simulink model "sm_tractor_row_crop"  (R2024b)
settings: Solver=ode23t  StartTime=0.0  StopTime=20  FixedStep=1/1000  MaxStep=0.2  RelTol=1e-3  AbsTol=1e-3  EnableMultiTasking=on
PostLoadFcn:
  | sm_tractor_row_crop_config_maneuver(bdroot,VehicleData,'stepsteer');
StartFcn:
  | tic
StopFcn:
  | Elapsed_Sim_Time = toc;
undefined symbols (not defined in the file): FL, FR, HMPST, InitVehicle, Maneuver, RL, RR, SceneData, targetSpeed, VehicleData, X, Y, Z
libraries: sm_lib x121, sm_vehicle_utilities_lib x41, fl_lib x15, nesl_utility x14, simulink x3, sm_tractor_row_crop_lib x3, sm_tractor_row_crop_lib_vnts x2, Driver_Long_Lat_Stanley x1, Maneuver_Get_Pose x1
(part 2 of 4)

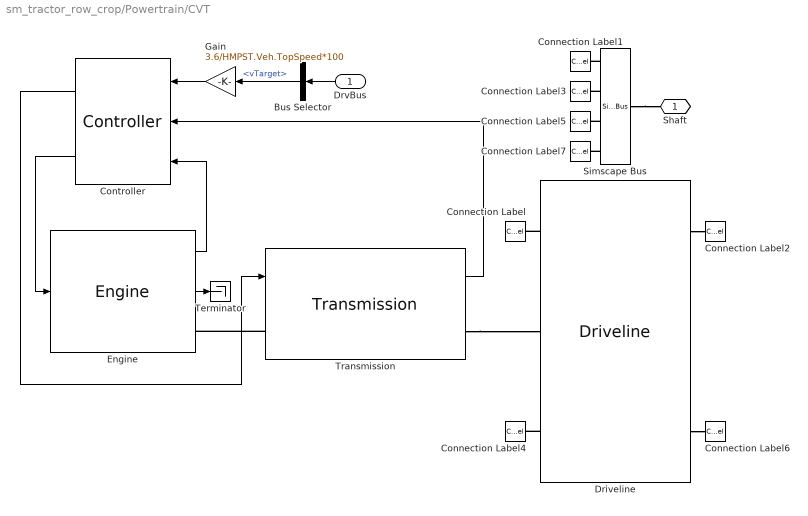
== system sm_tractor_row_crop/Powertrain/CVT ==
  DrvBus : Inport
  Bus Selector : BusSelector  OutputSignals=Reference.vTarget
  Connection Label : ConnectionLabel  Label=FL
  Connection Label1 : ConnectionLabel  Label=FL
  Connection Label2 : ConnectionLabel  Label=FR
  Connection Label3 : ConnectionLabel  Label=FR
  Connection Label4 : ConnectionLabel  Label=RL
  Connection Label5 : ConnectionLabel  Label=RL
  Connection Label6 : ConnectionLabel  Label=RR
  Connection Label7 : ConnectionLabel  Label=RR
  Controller : sm_tractor_row_crop_lib/Controller  SystemSampleTime=-1  VariantActivationTime=update diagram  AllowFlexibleInterface=on  Latency=0  AutoFrameSizeCalculation=off
  Driveline : sm_tractor_row_crop_lib/Driveline  SystemSampleTime=-1  VariantActivationTime=update diagram  AllowFlexibleInterface=on  Latency=0  AutoFrameSizeCalculation=off
  Engine : sm_tractor_row_crop_lib_vnts/Engine  SystemSampleTime=-1  VariantControl=Choice  LabelModeActiveChoice=Droop  VariantActivationTime=update diagram  AllowFlexibleInterface=on  Latency=0  AutoFrameSizeCalculation=off
      settings: AttributesFormatString=%<LabelModeActiveChoice>
  Gain : Gain  Gain=3.6/HMPST.Veh.TopSpeed*100
  Simscape Bus : SimscapeBus  HierarchyStrings=FL;FR;RL;RR
  Terminator : Terminator
  Transmission : sm_tractor_row_crop_lib_vnts/Transmission  SystemSampleTime=-1  VariantControl=Choice  LabelModeActiveChoice=Hydrostatic  VariantActivationTime=update diagram  AllowFlexibleInterface=on  Latency=0  AutoFrameSizeCalculation=off
      settings: AttributesFormatString=%<LabelModeActiveChoice>
  Shaft : PMIOPort  Side=Right
  wires:
  Engine/2 -> Terminator/1
  Transmission/1 -> Controller/2
  Controller/1 -> Transmission/1
  Controller/2 -> Engine/1
  Engine/1 -> Controller/3
  Bus Selector/1 -> Gain/1  "<vTarget>"
  Gain/1 -> Controller/1
  DrvBus/1 -> Bus Selector/1
  connections:
  Transmission/RConn1 -- Driveline/LConn2
  Simscape Bus/RConn1 -- Shaft/RConn1
  Transmission/LConn1 -- Engine/RConn1
  Simscape Bus/LConn2 -- Connection Label3/LConn1
  Simscape Bus/LConn1 -- Connection Label1/LConn1
  Simscape Bus/LConn4 -- Connection Label7/LConn1
  Simscape Bus/LConn3 -- Connection Label5/LConn1
  Driveline/LConn1 -- Connection Label4/LConn1
  Driveline/LConn3 -- Connection Label/LConn1
  Driveline/RConn1 -- Connection Label6/LConn1
  Driveline/RConn3 -- Connection Label2/LConn1

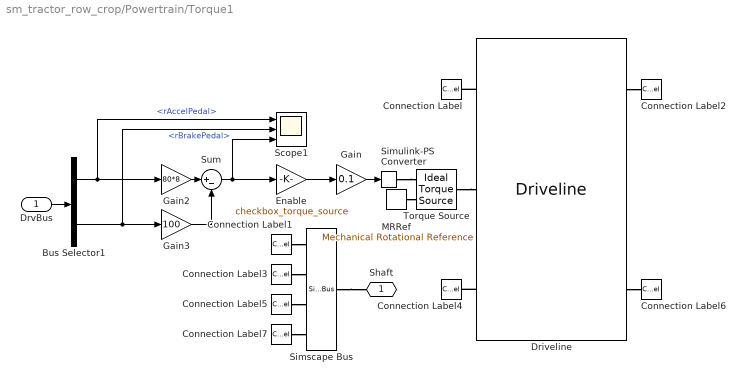
== system sm_tractor_row_crop/Powertrain/Torque1 ==
  DrvBus : Inport
  Bus Selector1 : BusSelector  OutputSignals=rAccelPedal,rBrakePedal
  Connection Label : ConnectionLabel  Label=FL
  Connection Label1 : ConnectionLabel  Label=FL
  Connection Label2 : ConnectionLabel  Label=FR
  Connection Label3 : ConnectionLabel  Label=FR
  Connection Label4 : ConnectionLabel  Label=RL
  Connection Label5 : ConnectionLabel  Label=RL
  Connection Label6 : ConnectionLabel  Label=RR
  Connection Label7 : ConnectionLabel  Label=RR
  Driveline : sm_tractor_row_crop_lib/Driveline  SystemSampleTime=-1  VariantActivationTime=update diagram  AllowFlexibleInterface=on  Latency=0  AutoFrameSizeCalculation=off
  Enable : Gain  Gain=checkbox_torque_source
  Gain : Gain  Gain=0.1
  Gain2 : Gain  Gain=80*8
  Gain3 : Gain  Gain=100
  MRRef : fl_lib/Mechanical/Rotational Elements/Mechanical Rotational Reference
  Scope1 : Scope  NumInputPorts=3
  Simscape Bus : SimscapeBus  HierarchyStrings=FL;FR;RL;RR
  Simulink-PS Converter : nesl_utility/Simulink-PS Converter  PhysicalDomain=network_engine_domain  SubClassName=ps_input  LeftPortType=input  RightPortType=output  PseudoPeriodic=off  Frequencies=[]  NoiseDistribution=none  NoiseParameters=[]  Unit=1  AffineConversion=off  FilteringAndDerivatives=provide  SimscapeFilterOrder=1  InputFilterTimeConstant=0.001  UdotUserProvided=0
  Sum : Sum  Inputs=|+-
  Torque Source : fl_lib/Mechanical/Mechanical Sources/Ideal Torque Source
  Shaft : PMIOPort  Side=Right
  wires:
  Sum/1 -> Scope1/3, Enable/1
  DrvBus/1 -> Bus Selector1/1
  Bus Selector1/2 -> Scope1/2, Gain3/1  "<rBrakePedal>"
  Gain3/1 -> Sum/2
  Gain2/1 -> Sum/1
  Bus Selector1/1 -> Scope1/1, Gain2/1  "<rAccelPedal>"
  Gain/1 -> Simulink-PS Converter/1
  Enable/1 -> Gain/1
  connections:
  Driveline/RConn3 -- Connection Label2/LConn1
  Driveline/LConn3 -- Connection Label/LConn1
  Driveline/RConn1 -- Connection Label6/LConn1
  Driveline/LConn1 -- Connection Label4/LConn1
  Simscape Bus/RConn1 -- Shaft/RConn1
  MRRef/LConn1 -- Torque Source/RConn2
  Torque Source/LConn1 -- Driveline/LConn2
  Simulink-PS Converter/RConn1 -- Torque Source/RConn1
  Connection Label1/LConn1 -- Simscape Bus/LConn1
  Connection Label3/LConn1 -- Simscape Bus/LConn2
  Connection Label5/LConn1 -- Simscape Bus/LConn3
  Connection Label7/LConn1 -- Simscape Bus/LConn4

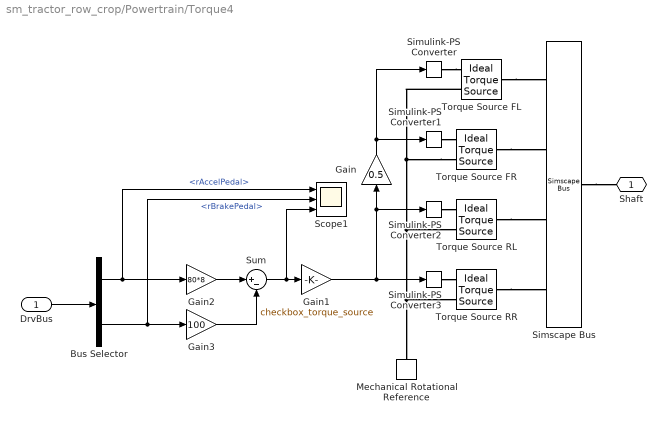
== system sm_tractor_row_crop/Powertrain/Torque4 ==
  DrvBus : Inport
  Bus Selector : BusSelector  OutputSignals=rAccelPedal,rBrakePedal
  Gain : Gain  Gain=0.5
  Gain1 : Gain  Gain=checkbox_torque_source
  Gain2 : Gain  Gain=80*8
  Gain3 : Gain  Gain=100
  Mechanical Rotational Reference : fl_lib/Mechanical/Rotational Elements/Mechanical Rotational Reference
  Scope1 : Scope  NumInputPorts=3
  Simscape Bus : SimscapeBus  HierarchyStrings=FL;FR;RL;RR
  Simulink-PS Converter{,1..3} (4 alike) : nesl_utility/Simulink-PS Converter  PhysicalDomain=network_engine_domain  SubClassName=ps_input  LeftPortType=input  RightPortType=output  PseudoPeriodic=off  Frequencies=[]  NoiseDistribution=none  NoiseParameters=[]  Unit=1  AffineConversion=off  FilteringAndDerivatives=provide  SimscapeFilterOrder=1  InputFilterTimeConstant=0.001  UdotUserProvided=0
  Sum : Sum  Inputs=|+-
  Torque Source FL : fl_lib/Mechanical/Mechanical Sources/Ideal Torque Source
  Torque Source FR : fl_lib/Mechanical/Mechanical Sources/Ideal Torque Source
  Torque Source RL : fl_lib/Mechanical/Mechanical Sources/Ideal Torque Source
  Torque Source RR : fl_lib/Mechanical/Mechanical Sources/Ideal Torque Source
  Shaft : PMIOPort  Side=Right
  wires:
  Bus Selector/1 -> Scope1/1, Gain2/1  "<rAccelPedal>"
  DrvBus/1 -> Bus Selector/1
  Sum/1 -> Scope1/3, Gain1/1
  Bus Selector/2 -> Scope1/2, Gain3/1  "<rBrakePedal>"
  Gain2/1 -> Sum/1
  Gain3/1 -> Sum/2
  Gain1/1 -> Simulink-PS Converter3/1, Simulink-PS Converter2/1, Gain/1
  Gain/1 -> Simulink-PS Converter1/1, Simulink-PS Converter/1
  connections:
  Torque Source FR/RConn2 -- Mechanical Rotational Reference/LConn1 -- Torque Source RR/RConn2 -- Torque Source RL/RConn2 -- Torque Source FL/RConn2
  Simulink-PS Converter3/RConn1 -- Torque Source RR/RConn1
  Simulink-PS Converter2/RConn1 -- Torque Source RL/RConn1
  Simulink-PS Converter1/RConn1 -- Torque Source FR/RConn1
  Simulink-PS Converter/RConn1 -- Torque Source FL/RConn1
  Torque Source RR/LConn1 -- Simscape Bus/LConn4
  Torque Source RL/LConn1 -- Simscape Bus/LConn3
  Torque Source FR/LConn1 -- Simscape Bus/LConn2
  Torque Source FL/LConn1 -- Simscape Bus/LConn1
  Simscape Bus/RConn1 -- Shaft/RConn1

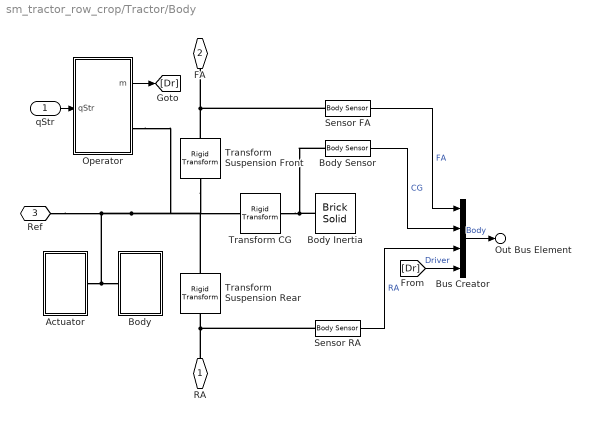
== system sm_tractor_row_crop/Tractor/Body ==
  qStr : Inport
  Actuator : Subsystem
  Body : Subsystem
  Body Inertia : sm_lib/Body Elements/Brick Solid  BrickDimensions=[0.1 0.1 0.1]  BrickDimensionsUnits=m  ExportEntireGeometry=off  InertiaType=Custom  BasedOnType=Density  Density=1000  DensityUnits=kg/(m^3)  Mass=mBody  MassUnits=kg  CenterOfMass=[0 0 0]  CenterOfMassUnits=m  MomentsOfInertia=JBody  MomentsOfInertiaUnits=kg*m^2  ProductsOfInertia=[0 0 0]  ProductsOfInertiaUnits=kg*m^2  GraphicType=FromGeometry  MarkerShape=Sphere  MarkerSize=10  GraphicVisPropType=SimpleVisualProperties  GraphicDiffuseColor=[0.4 0.6 1.0]  GraphicOpacity=1.0  GraphicSpecularColor=[0.5 0.5 0.5 1.0]  GraphicAmbientColor=[0.15 0.15 0.15 1.0]  GraphicEmissiveColor=[0.0 0.0 0.0 1.0]  GraphicShininess=75  DoExposeReferenceFrame=on  SerializedFrames=<Frames/>
  Body Sensor : sm_vehicle_utilities_lib/Body Sensor  offset_body_sensor=[0 0 0]
  Bus Creator : BusCreator  Inputs=4
  Operator : Subsystem  mask{popup_operator=None}
      mask prompts: popup_operator "Operator Type"
      mask init:
      | bh = gcb;
      | op_type = get_param(bh,'popup_operator');
      | switch op_type
      |     case 'None'
      |         set_param([bh '/Operator'],'popup_operator','None');
      |         set_param([bh '/Suspension'],'popup_suspension','None');
      |     case 'Human, Rigid Seat'
      |         set_param([bh '/Operator'],'popup_operator','Human');
      |         set_param([bh '/Suspension'],'popup_suspension','None');
      |     case 'Human, Suspension'
      |         set_param([bh '/Operator'],'popup_operator','Human');
      |         set_param([bh '/Suspension'],'popup_suspension','Heave Linear');
      | end
      settings: AttributesFormatString=%<popup_operator>
      mask TypeOptions popup_operator: None | Human, Rigid Seat | Human, Suspension
  Sensor FA : sm_vehicle_utilities_lib/Body Sensor  offset_body_sensor=[0 0 0]
  Sensor RA : sm_vehicle_utilities_lib/Body Sensor  offset_body_sensor=[0 0 0]
  Transform CG : sm_lib/Frames and Transforms/Rigid Transform  RotationMethod=None  FollAlignAxisA=+X  BaseAlignAxisA=+Y  FollAlignAxisB=+Y  BaseAlignAxisB=+Z  RotationStandardAxis=+Z  RotationAngle=0  RotationAngleUnits=deg  RotationArbitraryAxis=[0 0 1]  RotationSequenceAxes=FollowerAxes  RotationSequence=XYX  RotationSequenceAngles=[0 0 0]  RotationSequenceAnglesUnits=deg  RotationMatrix=[1 0 0; 0 1 0; 0 0 1]  Quaternion=[1 0 0 0]  TranslationMethod=Cartesian  TranslationCartesianOffset=xyzRefToCG  TranslationCartesianOffsetUnits=m  TranslationStandardAxis=+Z  TranslationStandardOffset=0  TranslationStandardOffsetUnits=m  TranslationROffset=0  TranslationROffsetUnits=m  TranslationThetaOffset=0  TranslationThetaOffsetUnits=deg  TranslationZOffset=0  TranslationZOffsetUnits=m
  Transform Suspension Front : sm_lib/Frames and Transforms/Rigid Transform  RotationMethod=None  FollAlignAxisA=+X  BaseAlignAxisA=+Y  FollAlignAxisB=+Y  BaseAlignAxisB=+Z  RotationStandardAxis=+Z  RotationAngle=0  RotationAngleUnits=deg  RotationArbitraryAxis=[0 0 1]  RotationSequenceAxes=FollowerAxes  RotationSequence=XYX  RotationSequenceAngles=[0 0 0]  RotationSequenceAnglesUnits=deg  RotationMatrix=[1 0 0; 0 1 0; 0 0 1]  Quaternion=[1 0 0 0]  TranslationMethod=StandardAxis  TranslationCartesianOffset=[0 0 0]  TranslationCartesianOffsetUnits=m  TranslationStandardAxis=+X  TranslationStandardOffset=xRefToFA  TranslationStandardOffsetUnits=m  TranslationROffset=0  TranslationROffsetUnits=m  TranslationThetaOffset=0  TranslationThetaOffsetUnits=deg  TranslationZOffset=0  TranslationZOffsetUnits=m
  Transform Suspension Rear : sm_lib/Frames and Transforms/Rigid Transform  RotationMethod=None  FollAlignAxisA=+X  BaseAlignAxisA=+Y  FollAlignAxisB=+Y  BaseAlignAxisB=+Z  RotationStandardAxis=+Z  RotationAngle=0  RotationAngleUnits=deg  RotationArbitraryAxis=[0 0 1]  RotationSequenceAxes=FollowerAxes  RotationSequence=XYX  RotationSequenceAngles=[0 0 0]  RotationSequenceAnglesUnits=deg  RotationMatrix=[1 0 0; 0 1 0; 0 0 1]  Quaternion=[1 0 0 0]  TranslationMethod=StandardAxis  TranslationCartesianOffset=[0 0 0]  TranslationCartesianOffsetUnits=m  TranslationStandardAxis=+X  TranslationStandardOffset=xRefToRA  TranslationStandardOffsetUnits=m  TranslationROffset=0  TranslationROffsetUnits=m  TranslationThetaOffset=0  TranslationThetaOffsetUnits=deg  TranslationZOffset=0  TranslationZOffsetUnits=m
  RA : PMIOPort  Side=Left
  FA : PMIOPort  Port=2  Side=Right
  Ref : PMIOPort  Port=3  Side=Right
  Out Bus Element : Outport  PortName=m  Element=Body
  wires:
  Body Sensor/1 -> Bus Creator/2  "CG"
  Sensor FA/1 -> Bus Creator/1  "FA"
  Sensor RA/1 -> Bus Creator/3  "RA"
  Bus Creator/1 -> Out Bus Element/1  "Body"
  [Dr] -> Bus Creator/4  "Driver"
  qStr/1 -> Operator/1(qStr)
  Operator/1(m) -> [Dr]
  connections:
  RA/RConn1 -- Transform Suspension Rear/RConn1 -- Sensor RA/LConn1
  Actuator/LConn1 -- Body/RConn1 -- Ref/RConn1 -- Operator/RConn1 -- Transform Suspension Front/LConn1 -- Transform Suspension Rear/LConn1 -- Transform CG/LConn1
  Transform Suspension Front/RConn1 -- FA/RConn1 -- Sensor FA/LConn1
  Transform CG/RConn1 -- Body Inertia/RConn1 -- Body Sensor/LConn1

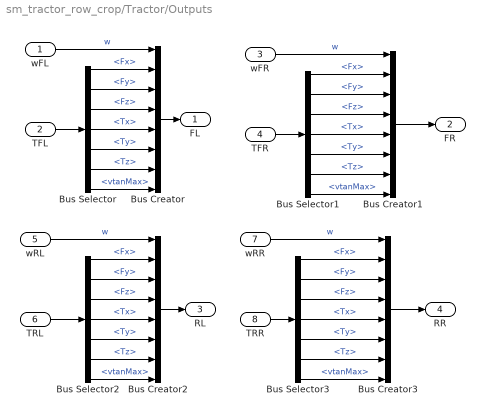
== system sm_tractor_row_crop/Tractor/Outputs ==
  wFL : Inport
  TFL : Inport  Port=2
  wFR : Inport  Port=3
  TFR : Inport  Port=4
  wRL : Inport  Port=5
  TRL : Inport  Port=6
  wRR : Inport  Port=7
  TRR : Inport  Port=8
  Bus Creator{,1..3} (4 alike) : BusCreator  Inputs=8
  Bus Selector{,1..3} (4 alike) : BusSelector  OutputSignals=Fx,Fy,Fz,Tx,Ty,Tz,vtanMax
  FL : Outport
  FR : Outport  Port=2
  RL : Outport  Port=3
  RR : Outport  Port=4
  wires:
  TFL/1 -> Bus Selector/1
  Bus Selector/1 -> Bus Creator/2  "<Fx>"
  Bus Selector/3 -> Bus Creator/4  "<Fz>"
  Bus Selector/4 -> Bus Creator/5  "<Tx>"
  wFL/1 -> Bus Creator/1  "w"
  Bus Selector/2 -> Bus Creator/3  "<Fy>"
  Bus Selector/6 -> Bus Creator/7  "<Tz>"
  Bus Selector/5 -> Bus Creator/6  "<Ty>"
  Bus Creator/1 -> FL/1
  Bus Creator1/1 -> FR/1
  Bus Selector1/5 -> Bus Creator1/6  "<Ty>"
  Bus Selector1/6 -> Bus Creator1/7  "<Tz>"
  Bus Selector1/2 -> Bus Creator1/3  "<Fy>"
  wFR/1 -> Bus Creator1/1  "w"
  Bus Selector1/4 -> Bus Creator1/5  "<Tx>"
  Bus Selector1/3 -> Bus Creator1/4  "<Fz>"
  Bus Selector1/1 -> Bus Creator1/2  "<Fx>"
  TFR/1 -> Bus Selector1/1
  TRR/1 -> Bus Selector3/1
  Bus Selector3/1 -> Bus Creator3/2  "<Fx>"
  Bus Selector3/3 -> Bus Creator3/4  "<Fz>"
  Bus Selector3/4 -> Bus Creator3/5  "<Tx>"
  wRR/1 -> Bus Creator3/1  "w"
  Bus Selector3/2 -> Bus Creator3/3  "<Fy>"
  Bus Selector3/6 -> Bus Creator3/7  "<Tz>"
  Bus Selector3/5 -> Bus Creator3/6  "<Ty>"
  Bus Creator3/1 -> RR/1
  Bus Creator2/1 -> RL/1
  Bus Selector2/5 -> Bus Creator2/6  "<Ty>"
  Bus Selector2/6 -> Bus Creator2/7  "<Tz>"
  Bus Selector2/2 -> Bus Creator2/3  "<Fy>"
  wRL/1 -> Bus Creator2/1  "w"
  Bus Selector2/4 -> Bus Creator2/5  "<Tx>"
  Bus Selector2/3 -> Bus Creator2/4  "<Fz>"
  Bus Selector2/1 -> Bus Creator2/2  "<Fx>"
  TRL/1 -> Bus Selector2/1
  Bus Selector/7 -> Bus Creator/8  "<vtanMax>"
  Bus Selector1/7 -> Bus Creator1/8  "<vtanMax>"
  Bus Selector2/7 -> Bus Creator2/8  "<vtanMax>"
  Bus Selector3/7 -> Bus Creator3/8  "<vtanMax>"

== system sm_tractor_row_crop/Tractor/Revolute Whl FL ==
  Mechanical Rotational Reference : fl_lib/Mechanical/Rotational Elements/Mechanical Rotational Reference
  Multibody-1D Interface : fl_lib/Mechanical/Multibody Interfaces/Rotational Multibody Interface
  PS-Simulink Converter : nesl_utility/PS-Simulink Converter  PhysicalDomain=network_engine_domain  SubClassName=ps_output  LeftPortType=input  RightPortType=output  PseudoPeriodic=off  Frequencies=[]  VectorFormat=inherit  Unit=inherit  AffineConversion=off
  Revolute Joint : sm_lib/Joints/Revolute Joint  JointMode=Normal  CompositeWrenchDir=FollowerOnBase  CompositeWrenchFrame=BaseFrame  SenseConstraintForce=off  SenseConstraintTorque=off  SenseTotalForce=off  SenseTotalTorque=off  PositionTargetSpecify=off  PositionTargetPriority=High  PositionTargetValue=0  PositionTargetValueUnits=deg  VelocityTargetSpecify=on  VelocityTargetPriority=High  VelocityTargetValue=initveh.Wheel.wFL  VelocityTargetValueUnits=rad/s  EquilibriumPosition=0  EquilibriumPositionUnits=rad  SpringStiffness=0  SpringStiffnessUnits=N*m/rad  DampingCoefficient=0  DampingCoefficientUnits=N*m/(rad/s)  LowerLimitSpecify=off  LowerLimitBound=-90  LowerLimitBoundUnits=deg  LowerLimitStiffness=1e4  LowerLimitStiffnessUnits=N*m/deg  LowerLimitDamping=10  LowerLimitDampingUnits=N*m/(deg/s)  LowerLimitTransitionRegionWidth=0.1  LowerLimitTransitionRegionWidthUnits=deg  UpperLimitSpecify=off  UpperLimitBound=90  UpperLimitBoundUnits=deg  UpperLimitStiffness=1e4  UpperLimitStiffnessUnits=N*m/deg  UpperLimitDamping=10  UpperLimitDampingUnits=N*m/(deg/s)  UpperLimitTransitionRegionWidth=0.1  UpperLimitTransitionRegionWidthUnits=deg  TorqueActuationMode=InputTorque  MotionActuationMode=ComputedMotion  SensePosition=off  SenseVelocity=on  SenseAcceleration=off  SenseTorqueForce=off  SenseLowerLimitTorqueForce=off  SenseUpperLimitTorqueForce=off
  B : PMIOPort  Side=Right
  R : PMIOPort  Port=2  Side=Left
  F : PMIOPort  Port=3  Side=Left
  Out Bus Element : Outport  PortName=m  Element=w
  wires:
  PS-Simulink Converter/1 -> Out Bus Element/1
  connections:
  Revolute Joint/LConn2 -- Multibody-1D Interface/LConn1
  Revolute Joint/RConn2 -- PS-Simulink Converter/LConn1 -- Multibody-1D Interface/RConn1
  F/RConn1 -- Revolute Joint/RConn1
  B/RConn1 -- Revolute Joint/LConn1
  Multibody-1D Interface/LConn2 -- Mechanical Rotational Reference/LConn1
  R/RConn1 -- Multibody-1D Interface/RConn2

== system sm_tractor_row_crop/Tractor/Revolute Whl FR ==
  Mechanical Rotational Reference : fl_lib/Mechanical/Rotational Elements/Mechanical Rotational Reference
  Multibody-1D Interface : fl_lib/Mechanical/Multibody Interfaces/Rotational Multibody Interface
  PS-Simulink Converter : nesl_utility/PS-Simulink Converter  PhysicalDomain=network_engine_domain  SubClassName=ps_output  LeftPortType=input  RightPortType=output  PseudoPeriodic=off  Frequencies=[]  VectorFormat=inherit  Unit=inherit  AffineConversion=off
  Revolute Joint : sm_lib/Joints/Revolute Joint  JointMode=Normal  CompositeWrenchDir=FollowerOnBase  CompositeWrenchFrame=BaseFrame  SenseConstraintForce=off  SenseConstraintTorque=off  SenseTotalForce=off  SenseTotalTorque=off  PositionTargetSpecify=off  PositionTargetPriority=High  PositionTargetValue=0  PositionTargetValueUnits=deg  VelocityTargetSpecify=on  VelocityTargetPriority=High  VelocityTargetValue=initveh.Wheel.wFR  VelocityTargetValueUnits=rad/s  EquilibriumPosition=0  EquilibriumPositionUnits=rad  SpringStiffness=0  SpringStiffnessUnits=N*m/rad  DampingCoefficient=0  DampingCoefficientUnits=N*m/(rad/s)  LowerLimitSpecify=off  LowerLimitBound=-90  LowerLimitBoundUnits=deg  LowerLimitStiffness=1e4  LowerLimitStiffnessUnits=N*m/deg  LowerLimitDamping=10  LowerLimitDampingUnits=N*m/(deg/s)  LowerLimitTransitionRegionWidth=0.1  LowerLimitTransitionRegionWidthUnits=deg  UpperLimitSpecify=off  UpperLimitBound=90  UpperLimitBoundUnits=deg  UpperLimitStiffness=1e4  UpperLimitStiffnessUnits=N*m/deg  UpperLimitDamping=10  UpperLimitDampingUnits=N*m/(deg/s)  UpperLimitTransitionRegionWidth=0.1  UpperLimitTransitionRegionWidthUnits=deg  TorqueActuationMode=InputTorque  MotionActuationMode=ComputedMotion  SensePosition=off  SenseVelocity=on  SenseAcceleration=off  SenseTorqueForce=off  SenseLowerLimitTorqueForce=off  SenseUpperLimitTorqueForce=off
  B : PMIOPort  Side=Right
  R : PMIOPort  Port=2  Side=Left
  F : PMIOPort  Port=3  Side=Left
  Out Bus Element : Outport  PortName=m  Element=w
  wires:
  PS-Simulink Converter/1 -> Out Bus Element/1
  connections:
  R/RConn1 -- Multibody-1D Interface/RConn2
  Multibody-1D Interface/LConn2 -- Mechanical Rotational Reference/LConn1
  B/RConn1 -- Revolute Joint/LConn1
  F/RConn1 -- Revolute Joint/RConn1
  PS-Simulink Converter/LConn1 -- Revolute Joint/RConn2 -- Multibody-1D Interface/RConn1
  Revolute Joint/LConn2 -- Multibody-1D Interface/LConn1

== system sm_tractor_row_crop/Tractor/Revolute Whl RL ==
  Mechanical Rotational Reference : fl_lib/Mechanical/Rotational Elements/Mechanical Rotational Reference
  Multibody-1D Interface : fl_lib/Mechanical/Multibody Interfaces/Rotational Multibody Interface
  PS-Simulink Converter : nesl_utility/PS-Simulink Converter  PhysicalDomain=network_engine_domain  SubClassName=ps_output  LeftPortType=input  RightPortType=output  PseudoPeriodic=off  Frequencies=[]  VectorFormat=inherit  Unit=inherit  AffineConversion=off
  Revolute Joint : sm_lib/Joints/Revolute Joint  JointMode=Normal  CompositeWrenchDir=FollowerOnBase  CompositeWrenchFrame=BaseFrame  SenseConstraintForce=off  SenseConstraintTorque=off  SenseTotalForce=off  SenseTotalTorque=off  PositionTargetSpecify=off  PositionTargetPriority=High  PositionTargetValue=0  PositionTargetValueUnits=deg  VelocityTargetSpecify=on  VelocityTargetPriority=High  VelocityTargetValue=initveh.Wheel.wRL  VelocityTargetValueUnits=rad/s  EquilibriumPosition=0  EquilibriumPositionUnits=rad  SpringStiffness=0  SpringStiffnessUnits=N*m/rad  DampingCoefficient=0  DampingCoefficientUnits=N*m/(rad/s)  LowerLimitSpecify=off  LowerLimitBound=-90  LowerLimitBoundUnits=deg  LowerLimitStiffness=1e4  LowerLimitStiffnessUnits=N*m/deg  LowerLimitDamping=10  LowerLimitDampingUnits=N*m/(deg/s)  LowerLimitTransitionRegionWidth=0.1  LowerLimitTransitionRegionWidthUnits=deg  UpperLimitSpecify=off  UpperLimitBound=90  UpperLimitBoundUnits=deg  UpperLimitStiffness=1e4  UpperLimitStiffnessUnits=N*m/deg  UpperLimitDamping=10  UpperLimitDampingUnits=N*m/(deg/s)  UpperLimitTransitionRegionWidth=0.1  UpperLimitTransitionRegionWidthUnits=deg  TorqueActuationMode=InputTorque  MotionActuationMode=ComputedMotion  SensePosition=off  SenseVelocity=on  SenseAcceleration=off  SenseTorqueForce=off  SenseLowerLimitTorqueForce=off  SenseUpperLimitTorqueForce=off
  B : PMIOPort  Side=Right
  R : PMIOPort  Port=2  Side=Left
  F : PMIOPort  Port=3  Side=Left
  Out Bus Element : Outport  PortName=m  Element=w
  wires:
  PS-Simulink Converter/1 -> Out Bus Element/1
  connections:
  R/RConn1 -- Multibody-1D Interface/RConn2
  Multibody-1D Interface/LConn2 -- Mechanical Rotational Reference/LConn1
  B/RConn1 -- Revolute Joint/LConn1
  F/RConn1 -- Revolute Joint/RConn1
  PS-Simulink Converter/LConn1 -- Revolute Joint/RConn2 -- Multibody-1D Interface/RConn1
  Revolute Joint/LConn2 -- Multibody-1D Interface/LConn1

== system sm_tractor_row_crop/Tractor/Revolute Whl RR ==
  Mechanical Rotational Reference : fl_lib/Mechanical/Rotational Elements/Mechanical Rotational Reference
  Multibody-1D Interface : fl_lib/Mechanical/Multibody Interfaces/Rotational Multibody Interface
  PS-Simulink Converter : nesl_utility/PS-Simulink Converter  PhysicalDomain=network_engine_domain  SubClassName=ps_output  LeftPortType=input  RightPortType=output  PseudoPeriodic=off  Frequencies=[]  VectorFormat=inherit  Unit=inherit  AffineConversion=off
  Revolute Joint : sm_lib/Joints/Revolute Joint  JointMode=Normal  CompositeWrenchDir=FollowerOnBase  CompositeWrenchFrame=BaseFrame  SenseConstraintForce=off  SenseConstraintTorque=off  SenseTotalForce=off  SenseTotalTorque=off  PositionTargetSpecify=off  PositionTargetPriority=High  PositionTargetValue=0  PositionTargetValueUnits=deg  VelocityTargetSpecify=on  VelocityTargetPriority=High  VelocityTargetValue=initveh.Wheel.wRR  VelocityTargetValueUnits=rad/s  EquilibriumPosition=0  EquilibriumPositionUnits=rad  SpringStiffness=0  SpringStiffnessUnits=N*m/rad  DampingCoefficient=0  DampingCoefficientUnits=N*m/(rad/s)  LowerLimitSpecify=off  LowerLimitBound=-90  LowerLimitBoundUnits=deg  LowerLimitStiffness=1e4  LowerLimitStiffnessUnits=N*m/deg  LowerLimitDamping=10  LowerLimitDampingUnits=N*m/(deg/s)  LowerLimitTransitionRegionWidth=0.1  LowerLimitTransitionRegionWidthUnits=deg  UpperLimitSpecify=off  UpperLimitBound=90  UpperLimitBoundUnits=deg  UpperLimitStiffness=1e4  UpperLimitStiffnessUnits=N*m/deg  UpperLimitDamping=10  UpperLimitDampingUnits=N*m/(deg/s)  UpperLimitTransitionRegionWidth=0.1  UpperLimitTransitionRegionWidthUnits=deg  TorqueActuationMode=InputTorque  MotionActuationMode=ComputedMotion  SensePosition=off  SenseVelocity=on  SenseAcceleration=off  SenseTorqueForce=off  SenseLowerLimitTorqueForce=off  SenseUpperLimitTorqueForce=off
  B : PMIOPort  Side=Right
  R : PMIOPort  Port=2  Side=Left
  F : PMIOPort  Port=3  Side=Left
  Out Bus Element : Outport  PortName=m  Element=w
  wires:
  PS-Simulink Converter/1 -> Out Bus Element/1
  connections:
  Revolute Joint/LConn2 -- Multibody-1D Interface/LConn1
  Multibody-1D Interface/RConn1 -- Revolute Joint/RConn2 -- PS-Simulink Converter/LConn1
  F/RConn1 -- Revolute Joint/RConn1
  B/RConn1 -- Revolute Joint/LConn1
  Multibody-1D Interface/LConn2 -- Mechanical Rotational Reference/LConn1
  R/RConn1 -- Multibody-1D Interface/RConn2

== system sm_tractor_row_crop/Tractor/Scene ==
  Flat : Subsystem  VariantControl=Flat
  Orchard : Subsystem  VariantControl=Orchard
  Plateau : Subsystem  VariantControl=Plateau
  Rough Road : Subsystem  VariantControl=Rough_Road
  Uneven Road : Subsystem  VariantControl=Uneven_Road
  GFL : PMIOPort  Side=Left
  GFR : PMIOPort  Port=2  Side=Left
  GRL : PMIOPort  Port=3  Side=Left
  GRR : PMIOPort  Port=4  Side=Left
  RFL : PMIOPort  Port=5  Side=Left
  RFR : PMIOPort  Port=6  Side=Left
  RRL : PMIOPort  Port=7  Side=Left
  RRR : PMIOPort  Port=8  Side=Left

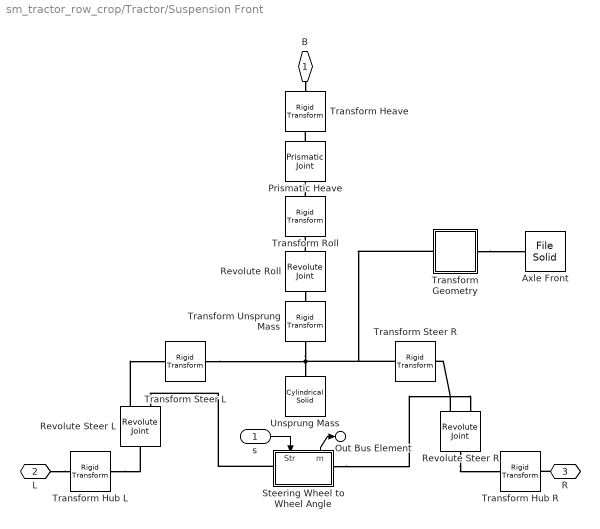
== system sm_tractor_row_crop/Tractor/Suspension Front ==
  s : Inport
  Axle Front : sm_lib/Body Elements/File Solid  ExtGeomFileName=Axle_Front.stl  UnitType=Custom  ExtGeomFileUnits=m  StepReaderType=HEX  ExportConvexHullGeometry=off  InertiaType=PointMass  BasedOnType=Density  Density=1000  DensityUnits=kg/m^3  Mass=0  MassUnits=kg  CenterOfMass=[0 0 0]  CenterOfMassUnits=m  MomentsOfInertia=[1 1 1]  MomentsOfInertiaUnits=kg*m^2  ProductsOfInertia=[0 0 0]  ProductsOfInertiaUnits=kg*m^2  GraphicType=FromGeometry  MarkerShape=Sphere  MarkerSize=10  GraphicVisPropType=SimpleVisualProperties  GraphicDiffuseColor=[0.8 0.8 0.8]  GraphicOpacity=1  GraphicSpecularColor=[0.5 0.5 0.5 1.0]  GraphicAmbientColor=[0.15 0.15 0.15 1.0]  GraphicEmissiveColor=[0.0 0.0 0.0 1.0]  GraphicShininess=75  DoExposeReferenceFrame=on  SerializedFrames=<Frames/>
  Prismatic Heave : sm_lib/Joints/Prismatic Joint  JointMode=Normal  CompositeWrenchDir=FollowerOnBase  CompositeWrenchFrame=BaseFrame  SenseConstraintForce=off  SenseConstraintTorque=off  SenseTotalForce=off  SenseTotalTorque=off  PositionTargetSpecify=off  PositionTargetPriority=High  PositionTargetValue=0  PositionTargetValueUnits=m  VelocityTargetSpecify=off  VelocityTargetPriority=High  VelocityTargetValue=0  VelocityTargetValueUnits=m/s  EquilibriumPosition=xEqHeave  EquilibriumPositionUnits=m  SpringStiffness=kHeave  SpringStiffnessUnits=N/m  DampingCoefficient=dHeave  DampingCoefficientUnits=N/(m/s)  LowerLimitSpecify=off  LowerLimitBound=-1  LowerLimitBoundUnits=m  LowerLimitStiffness=1e6  LowerLimitStiffnessUnits=N/m  LowerLimitDamping=1e3  LowerLimitDampingUnits=N/(m/s)  LowerLimitTransitionRegionWidth=1e-4  LowerLimitTransitionRegionWidthUnits=m  UpperLimitSpecify=off  UpperLimitBound=1  UpperLimitBoundUnits=m  UpperLimitStiffness=1e6  UpperLimitStiffnessUnits=N/m  UpperLimitDamping=1e3  UpperLimitDampingUnits=N/(m/s)  UpperLimitTransitionRegionWidth=1e-4  UpperLimitTransitionRegionWidthUnits=m  TorqueActuationMode=NoTorque  MotionActuationMode=ComputedMotion  SensePosition=off  SenseVelocity=off  SenseAcceleration=off  SenseTorqueForce=off  SenseLowerLimitTorqueForce=off  SenseUpperLimitTorqueForce=off
  Revolute Steer L : sm_lib/Joints/Revolute Joint  JointMode=Normal  CompositeWrenchDir=FollowerOnBase  CompositeWrenchFrame=BaseFrame  SenseConstraintForce=off  SenseConstraintTorque=off  SenseTotalForce=off  SenseTotalTorque=off  PositionTargetSpecify=off  PositionTargetPriority=High  PositionTargetValue=0  PositionTargetValueUnits=deg  VelocityTargetSpecify=off  VelocityTargetPriority=High  VelocityTargetValue=66  VelocityTargetValueUnits=rad/s  EquilibriumPosition=0  EquilibriumPositionUnits=rad  SpringStiffness=0  SpringStiffnessUnits=N*m/rad  DampingCoefficient=0  DampingCoefficientUnits=N*m/(rad/s)  LowerLimitSpecify=off  LowerLimitBound=-90  LowerLimitBoundUnits=deg  LowerLimitStiffness=1e4  LowerLimitStiffnessUnits=N*m/deg  LowerLimitDamping=10  LowerLimitDampingUnits=N*m/(deg/s)  LowerLimitTransitionRegionWidth=0.1  LowerLimitTransitionRegionWidthUnits=deg  UpperLimitSpecify=off  UpperLimitBound=90  UpperLimitBoundUnits=deg  UpperLimitStiffness=1e4  UpperLimitStiffnessUnits=N*m/deg  UpperLimitDamping=10  UpperLimitDampingUnits=N*m/(deg/s)  UpperLimitTransitionRegionWidth=0.1  UpperLimitTransitionRegionWidthUnits=deg  TorqueActuationMode=ComputedTorque  MotionActuationMode=InputMotion  SensePosition=off  SenseVelocity=off  SenseAcceleration=off  SenseTorqueForce=off  SenseLowerLimitTorqueForce=off  SenseUpperLimitTorqueForce=off
  Revolute Steer R : sm_lib/Joints/Revolute Joint  JointMode=Normal  CompositeWrenchDir=FollowerOnBase  CompositeWrenchFrame=BaseFrame  SenseConstraintForce=off  SenseConstraintTorque=off  SenseTotalForce=off  SenseTotalTorque=off  PositionTargetSpecify=off  PositionTargetPriority=High  PositionTargetValue=0  PositionTargetValueUnits=deg  VelocityTargetSpecify=off  VelocityTargetPriority=High  VelocityTargetValue=66  VelocityTargetValueUnits=rad/s  EquilibriumPosition=0  EquilibriumPositionUnits=rad  SpringStiffness=0  SpringStiffnessUnits=N*m/rad  DampingCoefficient=0  DampingCoefficientUnits=N*m/(rad/s)  LowerLimitSpecify=off  LowerLimitBound=-90  LowerLimitBoundUnits=deg  LowerLimitStiffness=1e4  LowerLimitStiffnessUnits=N*m/deg  LowerLimitDamping=10  LowerLimitDampingUnits=N*m/(deg/s)  LowerLimitTransitionRegionWidth=0.1  LowerLimitTransitionRegionWidthUnits=deg  UpperLimitSpecify=off  UpperLimitBound=90  UpperLimitBoundUnits=deg  UpperLimitStiffness=1e4  UpperLimitStiffnessUnits=N*m/deg  UpperLimitDamping=10  UpperLimitDampingUnits=N*m/(deg/s)  UpperLimitTransitionRegionWidth=0.1  UpperLimitTransitionRegionWidthUnits=deg  TorqueActuationMode=ComputedTorque  MotionActuationMode=InputMotion  SensePosition=off  SenseVelocity=off  SenseAcceleration=off  SenseTorqueForce=off  SenseLowerLimitTorqueForce=off  SenseUpperLimitTorqueForce=off
  Revolute Roll : sm_lib/Joints/Revolute Joint  JointMode=Normal  CompositeWrenchDir=FollowerOnBase  CompositeWrenchFrame=BaseFrame  SenseConstraintForce=off  SenseConstraintTorque=off  SenseTotalForce=off  SenseTotalTorque=off  PositionTargetSpecify=off  PositionTargetPriority=High  PositionTargetValue=0  PositionTargetValueUnits=deg  VelocityTargetSpecify=off  VelocityTargetPriority=High  VelocityTargetValue=0  VelocityTargetValueUnits=deg/s  EquilibriumPosition=aEqRoll  EquilibriumPositionUnits=rad  SpringStiffness=kRoll  SpringStiffnessUnits=N*m/rad  DampingCoefficient=dRoll  DampingCoefficientUnits=N*m/(rad/s)  LowerLimitSpecify=off  LowerLimitBound=-90  LowerLimitBoundUnits=deg  LowerLimitStiffness=1e4  LowerLimitStiffnessUnits=N*m/deg  LowerLimitDamping=10  LowerLimitDampingUnits=N*m/(deg/s)  LowerLimitTransitionRegionWidth=0.1  LowerLimitTransitionRegionWidthUnits=deg  UpperLimitSpecify=off  UpperLimitBound=90  UpperLimitBoundUnits=deg  UpperLimitStiffness=1e4  UpperLimitStiffnessUnits=N*m/deg  UpperLimitDamping=10  UpperLimitDampingUnits=N*m/(deg/s)  UpperLimitTransitionRegionWidth=0.1  UpperLimitTransitionRegionWidthUnits=deg  TorqueActuationMode=NoTorque  MotionActuationMode=ComputedMotion  SensePosition=off  SenseVelocity=off  SenseAcceleration=off  SenseTorqueForce=off  SenseLowerLimitTorqueForce=off  SenseUpperLimitTorqueForce=off
  Steering Wheel to Wheel Angle : Subsystem
      settings: PortSchema="{\"entries\":[{\"content\":{\"sides\":[{\"content\":{\"connectorIds\":[\"LConn1\"]},\"type\":\"ConnectorPlacement.EquallySpacedRectSide\",\"uuid\":\"65a6d75a-79bf-476b-9435-04bcf6c2ef18\"},{\"content\":{\"connectorIds\":[\"RConn1\"],\"side\":\"RIGHT\"},\"type\":\"ConnectorPlacement.EquallySpacedRectSide\",\"uuid\":\"4d91bb65-021e-4e19-8917-9509e9fd2683\"},{\"content\":{\"connectorIds\":[\"In1\",\"Out1\"],\"side\":\"TOP\"},\"type\":\"ConnectorPlacement.EquallySpacedRectSide\",\"uuid\":\"f7aac0ed-f2d6-4a01-9627-e78393360ed0\"}]},\"type\":\"ConnectorPlacement.EquallySpacedConnector\",\"uuid\":\"6c2d29d9-099e-4079-9b4f-de2c4ae6c2a7\"}],\"packageUris\":[\"http://schema.mathworks.com/mf0/Connector/R2020b\"],\"version\":\"1.0\"}"
  Transform Geometry : Subsystem
  Transform Heave : sm_lib/Frames and Transforms/Rigid Transform  RotationMethod=None  FollAlignAxisA=+X  BaseAlignAxisA=+Y  FollAlignAxisB=+Y  BaseAlignAxisB=+Z  RotationStandardAxis=+Z  RotationAngle=0.0  RotationAngleUnits=deg  RotationArbitraryAxis=[0 0 1]  RotationSequenceAxes=FollowerAxes  RotationSequence=XYX  RotationSequenceAngles=[0 0 0]  RotationSequenceAnglesUnits=deg  RotationMatrix=[1 0 0; 0 1 0; 0 0 1]  Quaternion=[1 0 0 0]  TranslationMethod=StandardAxis  TranslationCartesianOffset=[0 0 0]  TranslationCartesianOffsetUnits=m  TranslationStandardAxis=+Z  TranslationStandardOffset=zHeave  TranslationStandardOffsetUnits=m  TranslationROffset=0  TranslationROffsetUnits=m  TranslationThetaOffset=0  TranslationThetaOffsetUnits=deg  TranslationZOffset=0  TranslationZOffsetUnits=m
  Transform Hub L : sm_lib/Frames and Transforms/Rigid Transform  RotationMethod=StandardAxis  FollAlignAxisA=+X  BaseAlignAxisA=+Y  FollAlignAxisB=+Y  BaseAlignAxisB=+Z  RotationStandardAxis=-Y  RotationAngle=90  RotationAngleUnits=deg  RotationArbitraryAxis=[0 0 1]  RotationSequenceAxes=FollowerAxes  RotationSequence=XYX  RotationSequenceAngles=[0 0 0]  RotationSequenceAnglesUnits=deg  RotationMatrix=[1 0 0; 0 1 0; 0 0 1]  Quaternion=[1 0 0 0]  TranslationMethod=None  TranslationCartesianOffset=[0 0 0]  TranslationCartesianOffsetUnits=m  TranslationStandardAxis=+Z  TranslationStandardOffset=0  TranslationStandardOffsetUnits=m  TranslationROffset=0  TranslationROffsetUnits=m  TranslationThetaOffset=0  TranslationThetaOffsetUnits=deg  TranslationZOffset=0  TranslationZOffsetUnits=m
  Transform Hub R : sm_lib/Frames and Transforms/Rigid Transform  RotationMethod=StandardAxis  FollAlignAxisA=+X  BaseAlignAxisA=+Y  FollAlignAxisB=+Y  BaseAlignAxisB=+Z  RotationStandardAxis=-Y  RotationAngle=90  RotationAngleUnits=deg  RotationArbitraryAxis=[0 0 1]  RotationSequenceAxes=FollowerAxes  RotationSequence=XYX  RotationSequenceAngles=[0 0 0]  RotationSequenceAnglesUnits=deg  RotationMatrix=[1 0 0; 0 1 0; 0 0 1]  Quaternion=[1 0 0 0]  TranslationMethod=None  TranslationCartesianOffset=[0 0 0]  TranslationCartesianOffsetUnits=m  TranslationStandardAxis=+Z  TranslationStandardOffset=0  TranslationStandardOffsetUnits=m  TranslationROffset=0  TranslationROffsetUnits=m  TranslationThetaOffset=0  TranslationThetaOffsetUnits=deg  TranslationZOffset=0  TranslationZOffsetUnits=m
  Transform Roll : sm_lib/Frames and Transforms/Rigid Transform  RotationMethod=RotationSequence  FollAlignAxisA=+X  BaseAlignAxisA=+Y  FollAlignAxisB=+Y  BaseAlignAxisB=+Z  RotationStandardAxis=+Y  RotationAngle=90  RotationAngleUnits=deg  RotationArbitraryAxis=[0 0 1]  RotationSequenceAxes=FollowerAxes  RotationSequence=YZY  RotationSequenceAngles=[90 180 0]  RotationSequenceAnglesUnits=deg  RotationMatrix=[1 0 0; 0 1 0; 0 0 1]  Quaternion=[1 0 0 0]  TranslationMethod=StandardAxis  TranslationCartesianOffset=[0 0 0]  TranslationCartesianOffsetUnits=m  TranslationStandardAxis=+Z  TranslationStandardOffset=-zHeave+zRoll  TranslationStandardOffsetUnits=m  TranslationROffset=0  TranslationROffsetUnits=m  TranslationThetaOffset=0  TranslationThetaOffsetUnits=deg  TranslationZOffset=0  TranslationZOffsetUnits=m
  Transform Steer L : sm_lib/Frames and Transforms/Rigid Transform  RotationMethod=StandardAxis  FollAlignAxisA=+X  BaseAlignAxisA=+Y  FollAlignAxisB=+Y  BaseAlignAxisB=+Z  RotationStandardAxis=+Y  RotationAngle=90  RotationAngleUnits=deg  RotationArbitraryAxis=[0 0 1]  RotationSequenceAxes=FollowerAxes  RotationSequence=XYX  RotationSequenceAngles=[0 0 0]  RotationSequenceAnglesUnits=deg  RotationMatrix=[1 0 0; 0 1 0; 0 0 1]  Quaternion=[1 0 0 0]  TranslationMethod=Cartesian  TranslationCartesianOffset=[-zUnsprungMass+zHub 0 yTrack/2]  TranslationCartesianOffsetUnits=m  TranslationStandardAxis=+Z  TranslationStandardOffset=0  TranslationStandardOffsetUnits=m  TranslationROffset=0  TranslationROffsetUnits=m  TranslationThetaOffset=0  TranslationThetaOffsetUnits=deg  TranslationZOffset=0  TranslationZOffsetUnits=m
  Transform Steer R : sm_lib/Frames and Transforms/Rigid Transform  RotationMethod=StandardAxis  FollAlignAxisA=+X  BaseAlignAxisA=+Y  FollAlignAxisB=+Y  BaseAlignAxisB=+Z  RotationStandardAxis=+Y  RotationAngle=90  RotationAngleUnits=deg  RotationArbitraryAxis=[0 0 1]  RotationSequenceAxes=FollowerAxes  RotationSequence=XYX  RotationSequenceAngles=[0 0 0]  RotationSequenceAnglesUnits=deg  RotationMatrix=[1 0 0; 0 1 0; 0 0 1]  Quaternion=[1 0 0 0]  TranslationMethod=Cartesian  TranslationCartesianOffset=[-zUnsprungMass+zHub 0 -yTrack/2]  TranslationCartesianOffsetUnits=m  TranslationStandardAxis=+Z  TranslationStandardOffset=0  TranslationStandardOffsetUnits=m  TranslationROffset=0  TranslationROffsetUnits=m  TranslationThetaOffset=0  TranslationThetaOffsetUnits=deg  TranslationZOffset=0  TranslationZOffsetUnits=m
  Transform Unsprung Mass : sm_lib/Frames and Transforms/Rigid Transform  RotationMethod=StandardAxis  FollAlignAxisA=+X  BaseAlignAxisA=+Y  FollAlignAxisB=+Y  BaseAlignAxisB=+Z  RotationStandardAxis=+X  RotationAngle=90  RotationAngleUnits=deg  RotationArbitraryAxis=[0 0 1]  RotationSequenceAxes=FollowerAxes  RotationSequence=XYX  RotationSequenceAngles=[0 0 0]  RotationSequenceAnglesUnits=deg  RotationMatrix=[1 0 0; 0 1 0; 0 0 1]  Quaternion=[1 0 0 0]  TranslationMethod=StandardAxis  TranslationCartesianOffset=[0 0 0]  TranslationCartesianOffsetUnits=m  TranslationStandardAxis=+X  TranslationStandardOffset=-zRoll+zUnsprungMass  TranslationStandardOffsetUnits=m  TranslationROffset=0  TranslationROffsetUnits=m  TranslationThetaOffset=0  TranslationThetaOffsetUnits=deg  TranslationZOffset=0  TranslationZOffsetUnits=m
  Unsprung Mass : sm_lib/Body Elements/Cylindrical Solid  CylinderRadius=rUnsprungMass  CylinderRadiusUnits=m  CylinderLength=lUnsprungMass  CylinderLengthUnits=m  ExportEntireGeometry=off  InertiaType=Custom  BasedOnType=Density  Density=1000  DensityUnits=kg/(m^3)  Mass=mUnsprungMass  MassUnits=kg  CenterOfMass=[0 0 0]  CenterOfMassUnits=m  MomentsOfInertia=JUnsprungMass  MomentsOfInertiaUnits=kg*m^2  ProductsOfInertia=[0 0 0]  ProductsOfInertiaUnits=kg*m^2  GraphicType=FromGeometry  MarkerShape=Sphere  MarkerSize=10  GraphicVisPropType=SimpleVisualProperties  GraphicDiffuseColor=[0.6 0.6 0.6]  GraphicOpacity=0  GraphicSpecularColor=[0.5 0.5 0.5 1.0]  GraphicAmbientColor=[0.15 0.15 0.15 1.0]  GraphicEmissiveColor=[0.0 0.0 0.0 1.0]  GraphicShininess=75  DoExposeReferenceFrame=on  SerializedFrames=<Frames/>
  B : PMIOPort  Side=Left
  L : PMIOPort  Port=2  Side=Left
  R : PMIOPort  Port=3  Side=Right
  Out Bus Element : Outport  PortName=m  Element=Steer
  wires:
  s/1 -> Steering Wheel to Wheel Angle/1(Str)
  Steering Wheel to Wheel Angle/1(m) -> Out Bus Element/1
  connections:
  Transform Roll/LConn1 -- Prismatic Heave/RConn1
  Revolute Roll/LConn1 -- Transform Unsprung Mass/LConn1
  Prismatic Heave/LConn1 -- Transform Heave/RConn1
  Steering Wheel to Wheel Angle/LConn1 -- Revolute Steer L/LConn2
  Steering Wheel to Wheel Angle/RConn1 -- Revolute Steer R/LConn2
  B/RConn1 -- Transform Heave/LConn1
  Revolute Roll/RConn1 -- Transform Roll/RConn1
  L/RConn1 -- Transform Hub L/RConn1
  Transform Hub L/LConn1 -- Revolute Steer L/RConn1
  R/RConn1 -- Transform Hub R/RConn1
  Revolute Steer R/RConn1 -- Transform Hub R/LConn1
  Transform Steer L/LConn1 -- Transform Geometry/LConn1 -- Transform Steer R/LConn1 -- Transform Unsprung Mass/RConn1 -- Unsprung Mass/RConn1
  Revolute Steer R/LConn1 -- Transform Steer R/RConn1
  Revolute Steer L/LConn1 -- Transform Steer L/RConn1
  Transform Geometry/RConn1 -- Axle Front/RConn1
